simulink model "pid_controller"  (R2021b)
settings: Solver=FixedStepDiscrete  StartTime=0.0  StopTime=60  FixedStep=ts  RelTol=1e-3
undefined symbols (not defined in the file): kd, ki, kp, ts
settings Model: Creator=adish  LastModifiedBy=adish
settings OptimizationCC: DefaultParameterBehavior=Inlined  UseDivisionForNetSlopeComputation=on  GainParamInheritBuiltInType=on  UseFloatMulNetSlope=on  UseSpecifiedMinMax=on  InlineInvariantSignals=on  EnhancedBackFolding=on  BooleansAsBitfields=on  PassReuseOutputArgsAs=Individual arguments  StateBitsets=on  DataBitsets=on  ZeroExternalMemoryAtStartup=off  ZeroInternalMemoryAtStartup=off  NoFixptDivByZeroProtection=on  EfficientFloat2IntCast=on  LifeSpan=inf  OptimizeBlockOrder=speed  DifferentSizesBufferReuse=on  OptimizationPriority=RAM  EfficientTunableParamExpr=on
settings DebuggingCC: SignalInfNanChecking=warning  ReadBeforeWriteMsg=EnableAllAsError  WriteAfterWriteMsg=EnableAllAsError  WriteAfterReadMsg=EnableAllAsError  IntegerOverflowMsg=error  ParameterTunabilityLossMsg=error  UniqueDataStoreMsg=error  AssertControl=DisableAll  NonBusSignalsTreatedAsBus=error  SFInvalidInputDataAccessInChartInitDiag=error  SFTransitionOutsideNaturalParentDiag=error  SFUnreachableExecutionPathDiag=error  SFUndirectedBroadcastEventsDiag=error  IntegerSaturationMsg=error
settings HardwareCC: ProdLongLongMode=on
settings SFSimCC: CompileTimeRecursionLimit=0  EnableRuntimeRecursion=off  MATLABDynamicMemAlloc=off
settings RTWCC: Description=Embedded Coder  SystemTargetFile=ert.tlc  GenCodeOnly=on  TemplateMakefile=ert_default_tmf  GenerateReport=on  BuildConfiguration=Faster Runs  IncludeHyperlinkInReport=on  LaunchReport=on  GenerateTraceInfo=on  GenerateTraceReport=on  GenerateTraceReportSl=on  GenerateTraceReportSf=on  GenerateTraceReportEml=on  GenerateWebview=on  GenerateCodeMetricsReport=on  GenerateCodeReplacementReport=on
settings CodeAppCC: ForceParamTrailComments=on  IgnoreCustomStorageClasses=off  OperatorAnnotations=on  SimulinkDataObjDesc=on  SFDataObjDesc=on  MATLABFcnDesc=on  InsertBlockDesc=on  StateflowObjectComments=on  MATLABSourceComments=on  EnableCustomComments=on  ReqsInCode=on
settings ERTTargetCC: TargetLangStandard=C99 (ISO)  UtilityFuncGeneration=Shared location  GenerateSampleERTMain=on  CombineSignalStateStructs=on  SuppressErrorStatus=on  SupportNonFinite=off  ParenthesesLevel=Maximum  CastingMode=Standards  GenerateSharedConstants=off  InlinedParameterPlacement=NonHierarchical  ERTCustomFileTemplate=example_file_process.tlc  EnableSignedLeftShifts=off  EnableSignedRightShifts=off
settings ConfigComp: CovEnable=on  RecordCoverage=on  CovMetricSettings=dcmwe  CovModelRefEnable=on

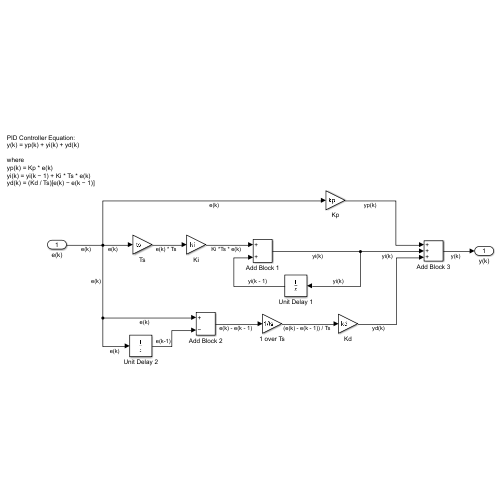
[thumbnail: Simulink's stored preview of the top-level diagram]
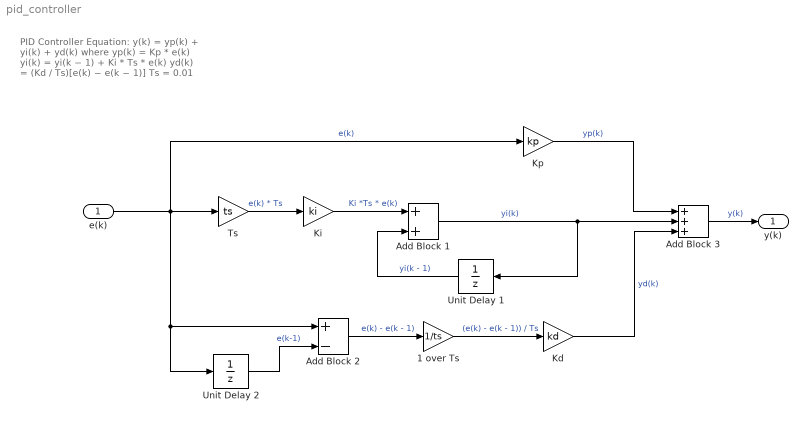
== system pid_controller ==
  note: PID Controller Equation:
      | y(k) = yp(k) + yi(k) + yd(k)
      |
      | where
      | yp(k) = Kp * e(k)
      | yi(k) = yi(k − 1) + Ki * Ts * e(k)
      | yd(k) = (Kd / Ts)[e(k) − e(k − 1)]
      | Ts = 0.01
  e(k) : Inport
  1 over Ts : Gain  Gain=1/ts
  Add Block 1 : Sum
  Add Block 2 : Sum  Inputs=+-
  Add Block 3 : Sum  Inputs=+++
  Kd : Gain  Gain=kd
  Ki : Gain  Gain=ki
  Kp : Gain  Gain=kp
  Ts : Gain  Gain=ts
  Unit Delay 1 : UnitDelay  SampleTime=0.01  HasFrameUpgradeWarning=on
  Unit Delay 2 : UnitDelay  SampleTime=0.01  HasFrameUpgradeWarning=on
  y(k) : Outport
  wires:
  Kp/1 -> Add Block 3/1  "yp(k)"
  Kd/1 -> Add Block 3/3  "yd(k)"
  Ki/1 -> Add Block 1/1  "Ki *Ts * e(k)"
  Unit Delay 1/1 -> Add Block 1/2  "yi(k - 1)"
  Ts/1 -> Ki/1  "e(k) * Ts"
  Add Block 3/1 -> y(k)/1  "y(k)"
  Add Block 1/1 -> Unit Delay 1/1, Add Block 3/2  "yi(k)"
  1 over Ts/1 -> Kd/1  "(e(k) - e(k - 1)) / Ts"
  Add Block 2/1 -> 1 over Ts/1  "e(k) - e(k - 1)"
  Unit Delay 2/1 -> Add Block 2/2  "e(k-1)"
  e(k)/1 -> Kp/1, Ts/1, Unit Delay 2/1, Add Block 2/1  "e(k)"
